simulink model "feedback_config"  (R2022a)
settings: Solver=VariableStepAuto  StartTime=0.0  StopTime=10.0  RelTol=1e-3
libraries: cstblocks x4
settings Model: Creator=WaineJunior  LastModifiedBy=WaineJunior

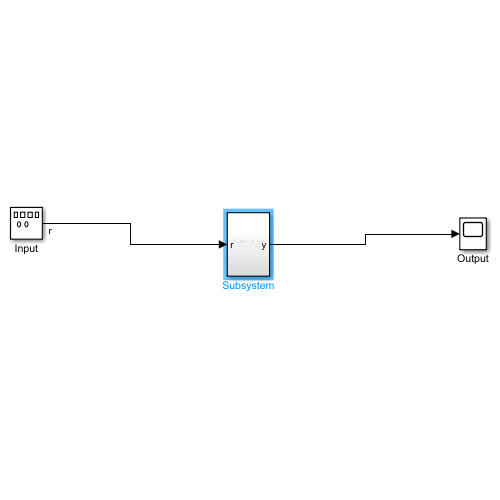
[thumbnail: Simulink's stored preview of the top-level diagram]
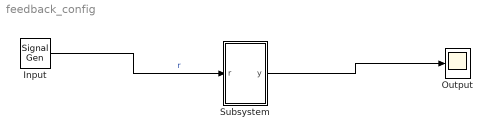
== system feedback_config ==
  Input : SignalGenerator
  Output : Scope
  Subsystem : Subsystem
  wires:
  Input/1 -> Subsystem/1(r)  "r"
  Subsystem/1(y) -> Output/1

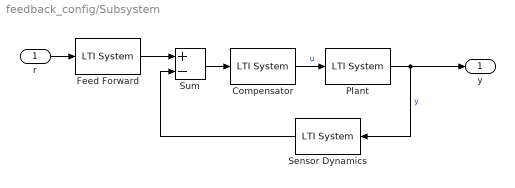
== system feedback_config/Subsystem ==
  r : Inport
  Compensator : cstblocks/LTI System  sys=C  IC=[]
  Feed Forward : cstblocks/LTI System  sys=F  IC=[]
  Plant : cstblocks/LTI System  sys=G  IC=[]
  Sensor Dynamics : cstblocks/LTI System  sys=H  IC=[]
  Sum : Sum  Inputs=+-
  y : Outport
  wires:
  Compensator/1 -> Plant/1  "u"
  Feed Forward/1 -> Sum/1
  Sensor Dynamics/1 -> Sum/2
  Plant/1 -> y/1, Sensor Dynamics/1  "y"
  Sum/1 -> Compensator/1
  r/1 -> Feed Forward/1
